simulink model "impuls_1"  (Simulink 7.6)
settings: Solver=ode45  StartTime=0.0  StopTime=2  RelTol=1e-3
values from neighbouring files (symbols this model uses):
  T_n = 127    [koef.m]
  T_v = 12.7    [koef.m]
settings Model: Creator=Johannes  LastModifiedBy=Johannes

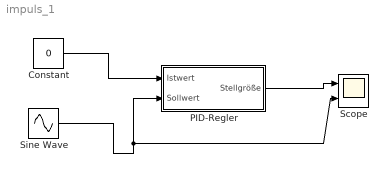
== system impuls_1 ==
  Constant : Constant  Value=0
  PID-Regler : Subsystem
  Scope : Scope  NumInputPorts=2
      settings: TimeRange=0.8000000000000002  YMin=-5~-3.75632911392405  YMax=5~0.2436708860759502  SampleInput=on  SampleTime=0.001
  Sine Wave : Sin  Frequency=4  SampleTime=0
  wires:
  Sine Wave/1 -> PID-Regler/2(Sollwert), Scope/2
  PID-Regler/1(Stellgröße) -> Scope/1
  Constant/1 -> PID-Regler/1(Istwert)

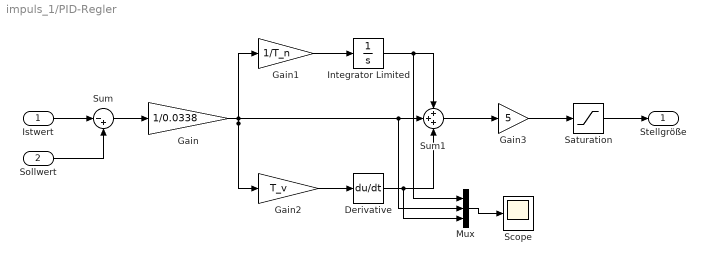
== system impuls_1/PID-Regler ==
  Istwert : Inport
  Sollwert : Inport  Port=2
  Derivative : Derivative
  Gain : Gain  Gain=1/0.0338
  Gain1 : Gain  Gain=1/T_n
  Gain2 : Gain  Gain=T_v
  Gain3 : Gain  Gain=5
  Integrator Limited : Integrator  LimitOutput=on  UpperSaturationLimit=10  LowerSaturationLimit=0
  Mux : Mux  Inputs=3
  Saturation : Saturate  UpperLimit=10  LowerLimit=0
  Scope : Scope
      settings: SampleInput=on  SampleTime=0.001
  Sum : Sum  Inputs=|-+
  Sum1 : Sum  Inputs=+++
  Stellgröße : Outport
  wires:
  Istwert/1 -> Sum/1
  Sollwert/1 -> Sum/2
  Sum/1 -> Gain/1
  Gain/1 -> Gain1/1, Gain2/1, Sum1/2, Mux/2
  Gain2/1 -> Derivative/1
  Gain1/1 -> Integrator Limited/1
  Integrator Limited/1 -> Sum1/1, Mux/1
  Derivative/1 -> Sum1/3, Mux/3
  Sum1/1 -> Gain3/1
  Gain3/1 -> Saturation/1
  Mux/1 -> Scope/1
  Saturation/1 -> Stellgröße/1
